simulink model "Ctrl_For_HRV_2026_6_22_codex"  (R2024b)
settings: Solver=ode4  StartTime=0.0  StopTime=100  FixedStep=0.02  RelTol=1e-3
InitFcn:
  | Parameter;
undefined symbols (not defined in the file or in its folder): CCI_DUI_AngleRate_Controller, CCI_DUI_FlowAngle_Controller, earth_r, fhan, g0, h_alpha, h_beta, h_miu, h_p, h_q, h_r, m, PNG_2026_6_3, r_alpha, r_beta, r_miu, r_p, r_q, r_r, S, xishu, xishu_D_0, xishu_L_0, xishu_l_0, xishu_m_0, xishu_n_0, xishu_Y_0
libraries: simulink x12
(part 2 of 2)

== matlab function Ctrl_For_HRV_2026_6_22_codex/MATLAB Function2 ==
  data: rM input; alphaCmd output; vM input; rT input; vT input; N input; maxLoadFactor input; g0 input; Q input; mass input; refArea input; alphaLimit input; bankCmd output; nNormalCmd output; nLateralCmd output; aCmd output; aCmdRaw output; lambda output; Vc output; omegaLOS output; Ma input
function [alphaCmd, bankCmd, nNormalCmd, nLateralCmd, aCmd, aCmdRaw, ...
    lambda, Vc, omegaLOS] = pnOverloadCommand3D(rM, vM, rT, vT, N, ...
    maxLoadFactor, g0, Q, mass, refArea, alphaLimit,Ma)
% pnOverloadCommand3D Vector PN guidance converted to alpha/bank commands.
%#codegen
%
% This function is intended for a Simulink MATLAB Function block.
%
% Inputs:
%   rM, vM          Vehicle position and velocity, 3-by-1, inertial frame
%   rT, vT          Target position and velocity, 3-by-1, inertial frame
%   N               Navigation constant
%   maxLoadFactor   Total overload limit [g]
%   g0              Standard gravity [m/s^2]
%   rho             Atmospheric density at current altitude [kg/m^3]
%   mass            Vehicle mass [kg]
%   refArea         Aerodynamic reference area [m^2]
%   CL0             Lift coefficient at alpha = 0
%   CLalpha         Lift-curve slope [1/rad]
%   alphaLimit      Absolute angle-of-attack limit [rad]
%
% Outputs:
%   alphaCmd        Angle-of-attack command [rad]
%   bankCmd         Bank-angle command [rad]
%   nNormalCmd      Signed normal overload command [g]
%   nLateralCmd     Signed lateral overload command [g]
%   aCmd            Limited acceleration command in inertial frame [m/s^2]
%   aCmdRaw         Raw PN acceleration before projection and limiting [m/s^2]
%   lambda          LOS unit vector
%   Vc              Closing velocity [m/s]
%   omegaLOS        LOS angular velocity vector [rad/s]
%
% Velocity-frame axis definition:
%   eForward        Along vehicle velocity
%   eLateral        Right side, perpendicular to forward and inertial up
%   eNormal         Positive upward in the velocity-vertical plane
%
% Command convention:
%   bankCmd = 0        Lift points along +eNormal
%   bankCmd > 0        Lift rotates from +eNormal toward +eLateral
%   alphaCmd > 0       Produces positive lift coefficient in the model

    r = rT - rM;
    v = vT - vM;
    R = norm(r);

    if R < 1e-9
        lambda = [1; 0; 0];
        Vc = 0;
        omegaLOS = [0; 0; 0];
        aCmdRaw = [0; 0; 0];
        aCmd = [0; 0; 0];
        alphaCmd = 0;
        bankCmd = 0;
        nNormalCmd = 0;
        nLateralCmd = 0;
        return;
    end

    lambda = r / R;
    Vc = -dot(r, v) / R;
    omegaLOS = cross(r, v) / R^2;

    if Vc > 0
        aCmdRaw = N * Vc * cross(omegaLOS, lambda);
    else
        aCmdRaw = [0; 0; 0];
    end

    [eForward, eNormal, eLateral] = velocityFrameAxes(vM);

    % Only the acceleration perpendicular to velocity is realizable as
    % normal/lateral overload command in this baseline model.
    aCmdNoAxial = aCmdRaw - dot(aCmdRaw, eForward) * eForward;
    aCmd = limitVectorMagnitude(aCmdNoAxial, maxLoadFactor * g0);

    nNormalCmd = dot(aCmd, eNormal) / g0;
    nLateralCmd = dot(aCmd, eLateral) / g0;

    [alphaCmd, bankCmd] = overloadToAlphaBank(nNormalCmd, nLateralCmd, ...
        vM, Q, mass, refArea, alphaLimit, g0);
end

function [alphaCmd, bankCmd] = overloadToAlphaBank(nNormalCmd, nLateralCmd, ...
     Q, mass, refArea, CLalpha, alphaLimit, g0,Ma)
% overloadToAlphaBank Convert velocity-frame overload to alpha and bank.
%
% The lift vector is assumed perpendicular to velocity:
%
%   nNormalCmd  = nLiftCmd * cos(bankCmd)
%   nLateralCmd = nLiftCmd * sin(bankCmd)
%
% The angle of attack is obtained from the simple aerodynamic model:
%
%   L = qbar * refArea * CL
%   CL = CL0 + CLalpha * alpha
%
% Replace this function with aerodynamic-table interpolation if your
% Simulink model has Mach/altitude-dependent CL(alpha, Mach, h).

    nLiftCmd = hypot(nNormalCmd, nLateralCmd);

    if nLiftCmd < 1e-9
        bankCmd = 0;
    else
        bankCmd = atan2(nLateralCmd, nNormalCmd);
    end


    if Q <= 1e-9 || refArea <= 0 || mass <= 0 || abs(CLalpha) <= 1e-9
        alphaCmd = 0;
        return;
    end

    CLRequired = nLiftCmd * mass * g0 / (Q * refArea);

    CL_func = @(alpha_deg) (-8.19e-2)+(4.7e-2)*Ma+(1.86e-2)*alpha_deg-(4.73e-4)*(alpha_deg*Ma)-(9.19e-3)*Ma^2-(1.52e-4)*alpha_deg^2+(5.99e-7)*(alpha_deg*Ma)^2+(7.74e-4)*Ma^3+(4.08e-6)*alpha_deg^3-(2.93e-5)*Ma^4+(4.12e-7)*Ma^5;
    alpha_cmd = fzero(@(a) CL_func(a) - CLRequired, [-alphaLimit, alphaLimit]);

    alphaCmd = min(max(alpha_cmd, -alphaLimit), alphaLimit);
end

function [eForward, eNormal, eLateral] = velocityFrameAxes(vM)
% velocityFrameAxes Build the velocity coordinate frame.

    speed = norm(vM);
    if speed < 1e-9
        eForward = [1; 0; 0];
    else
        eForward = vM / speed;
    end

    inertialUp = [0; 0; 1];
    eLateral = cross(inertialUp, eForward);

    if norm(eLateral) < 1e-9
        inertialRight = [0; 1; 0];
        eLateral = cross(inertialRight, eForward);
    end

    eLateral = eLateral / norm(eLateral);
    eNormal = cross(eForward, eLateral);
    eNormal = eNormal / norm(eNormal);
end

function y = limitVectorMagnitude(x, maxMagnitude)
% limitVectorMagnitude Saturate vector magnitude while preserving direction.

    xNorm = norm(x);
    if xNorm > maxMagnitude && xNorm > 0
        y = x * (maxMagnitude / xNorm);
    else
        y = x;
    end
end
